simulink model "PositionandSpeedCalculationComponent"  (R2025b)
settings: Solver=FixedStepDiscrete  StartTime=0.0  StopTime=10.0  RelTol=1e-3
settings Model: DataDictionary=TractionEmotorSoftwareArchInterfaceData.sldd  Creator=dakaihu  LastModifiedBy=dakaihu
settings OptimizationCC: ReuseModelBlockBuffer=off
settings RTWCC: GPUComputeCapability=3.5

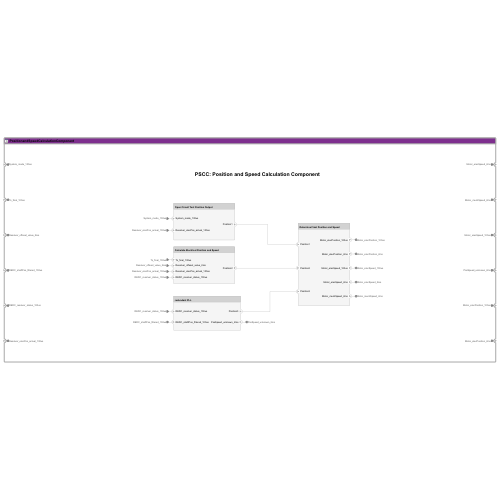
[thumbnail: Simulink's stored preview of the top-level diagram]
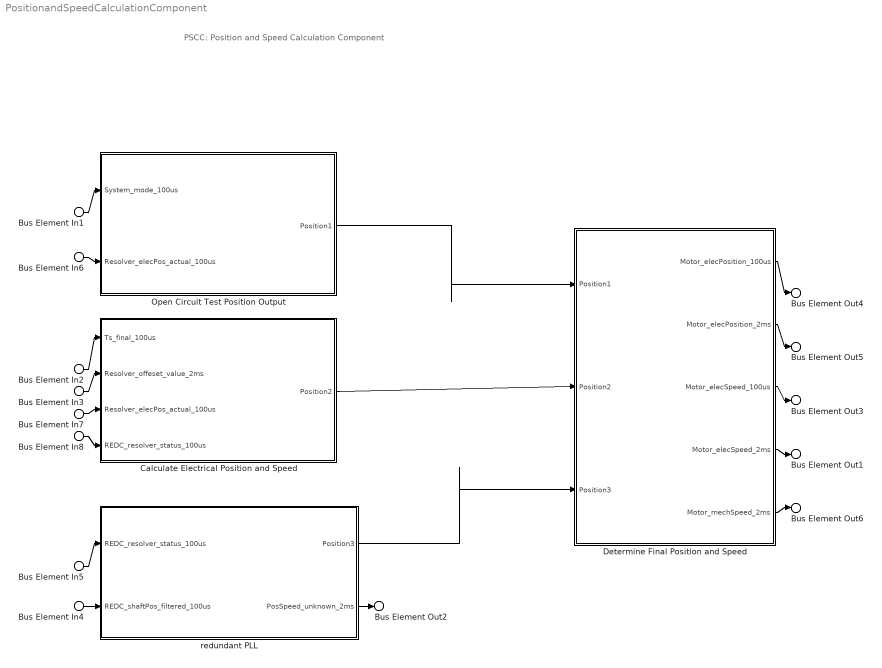
== system PositionandSpeedCalculationComponent ==
  note: PSCC: Position and Speed Calculation Component
  Bus Element In1 : Inport  PortName=System_mode_100us
  Bus Element In2 : Inport  Port=2  PortName=Ts_final_100us
  Bus Element In3 : Inport  Port=3  PortName=Resolver_offeset_value_2ms
  Bus Element In4 : Inport  Port=4  PortName=REDC_shaftPos_filtered_100us
  Bus Element In5 : Inport  Port=5  PortName=REDC_resolver_status_100us
  Bus Element In8 : Inport  Port=5  PortName=REDC_resolver_status_100us
  Bus Element In6 : Inport  Port=6  PortName=Resolver_elecPos_actual_100us
  Bus Element In7 : Inport  Port=6  PortName=Resolver_elecPos_actual_100us
  Calculate Electrical Position and Speed : Subsystem
      settings: PortSchema="{\"entries\":[{\"content\":{\"headerSize\":26,\"margin\":15,\"minimumSpacing\":25,\"sides\":[{\"content\":{\"connectorIds\":[\"In1\",\"In2\",\"In3\",\"In4\"]},\"type\":\"ConnectorPlacement.EquallySpacedRectSide\",\"uuid\":\"b16d0344-473b-4e33-95de-addbcbf18312\"},{\"content\":{\"connectorIds\":[\"Out1\"],\"side\":\"RIGHT\"},\"type\":\"ConnectorPlacement.EquallySpacedRectSide\",\"uuid\":\"7a9166db-696c-4525-87dc-5b08a993a34a\"},{\"content\":{\"connectorIds\":[],\"side\":\"TOP\"},\"type\":\"ConnectorPlacement.EquallySpacedRectSide\",\"uuid\":\"c2a34d16-9517-4bb1-8272-822cdcb4c574\"},{\"content\":{\"connectorIds\":[],\"side\":\"BOTTOM\"},\"type\":\"ConnectorPlacement.EquallySpacedRectSide\",\"uuid\":\"6a225a83-03bd-45b2-94f6-40f1b6cfb673\"}]},\"type\":\"ConnectorPlacement.EquallySpacedConnector\",\"uuid\":\"b21d167c-028b-4471-80b0-68b474506654\"}],\"packageUris\":[\"http://schema.mathworks.com/mf0/Connector/R2020b\"],\"version\":\"1.0\"}"
  Determine Final Position and Speed : Subsystem
      settings: PortSchema="{\"entries\":[{\"content\":{\"headerSize\":26,\"margin\":15,\"minimumSpacing\":25,\"sides\":[{\"content\":{\"connectorIds\":[\"In1\",\"In2\",\"In3\"]},\"type\":\"ConnectorPlacement.EquallySpacedRectSide\",\"uuid\":\"b16d0344-473b-4e33-95de-addbcbf18312\"},{\"content\":{\"connectorIds\":[\"Out1\",\"Out2\",\"Out3\",\"Out4\",\"Out5\"],\"side\":\"RIGHT\"},\"type\":\"ConnectorPlacement.EquallySpacedRectSide\",\"uuid\":\"7a9166db-696c-4525-87dc-5b08a993a34a\"},{\"content\":{\"connectorIds\":[],\"side\":\"TOP\"},\"type\":\"ConnectorPlacement.EquallySpacedRectSide\",\"uuid\":\"c2a34d16-9517-4bb1-8272-822cdcb4c574\"}]},\"type\":\"ConnectorPlacement.EquallySpacedConnector\",\"uuid\":\"b21d167c-028b-4471-80b0-68b474506654\"}],\"packageUris\":[\"http://schema.mathworks.com/mf0/Connector/R2020b\"],\"version\":\"1.0\"}"
  Open Circuit Test Position Output : Subsystem
      settings: PortSchema="{\"entries\":[{\"content\":{\"headerSize\":26,\"margin\":15,\"minimumSpacing\":25,\"sides\":[{\"content\":{\"connectorIds\":[\"In1\",\"In2\"]},\"type\":\"ConnectorPlacement.EquallySpacedRectSide\",\"uuid\":\"b16d0344-473b-4e33-95de-addbcbf18312\"},{\"content\":{\"connectorIds\":[\"Out1\"],\"side\":\"RIGHT\"},\"type\":\"ConnectorPlacement.EquallySpacedRectSide\",\"uuid\":\"7a9166db-696c-4525-87dc-5b08a993a34a\"},{\"content\":{\"connectorIds\":[],\"side\":\"TOP\"},\"type\":\"ConnectorPlacement.EquallySpacedRectSide\",\"uuid\":\"c2a34d16-9517-4bb1-8272-822cdcb4c574\"}]},\"type\":\"ConnectorPlacement.EquallySpacedConnector\",\"uuid\":\"b21d167c-028b-4471-80b0-68b474506654\"}],\"packageUris\":[\"http://schema.mathworks.com/mf0/Connector/R2020b\"],\"version\":\"1.0\"}"
  redundant PLL : Subsystem
      settings: PortSchema="{\"entries\":[{\"content\":{\"headerSize\":26,\"margin\":15,\"minimumSpacing\":25,\"sides\":[{\"content\":{\"connectorIds\":[\"In1\",\"In2\"]},\"type\":\"ConnectorPlacement.EquallySpacedRectSide\",\"uuid\":\"b16d0344-473b-4e33-95de-addbcbf18312\"},{\"content\":{\"connectorIds\":[\"Out1\",\"Out2\"],\"side\":\"RIGHT\"},\"type\":\"ConnectorPlacement.EquallySpacedRectSide\",\"uuid\":\"7a9166db-696c-4525-87dc-5b08a993a34a\"},{\"content\":{\"connectorIds\":[],\"side\":\"TOP\"},\"type\":\"ConnectorPlacement.EquallySpacedRectSide\",\"uuid\":\"c2a34d16-9517-4bb1-8272-822cdcb4c574\"}]},\"type\":\"ConnectorPlacement.EquallySpacedConnector\",\"uuid\":\"b21d167c-028b-4471-80b0-68b474506654\"}],\"packageUris\":[\"http://schema.mathworks.com/mf0/Connector/R2020b\"],\"version\":\"1.0\"}"
  Bus Element Out1 : Outport  PortName=Motor_elecSpeed_2ms
  Bus Element Out6 : Outport  Port=2  PortName=Motor_mechSpeed_2ms
  Bus Element Out3 : Outport  Port=3  PortName=Motor_elecSpeed_100us
  Bus Element Out2 : Outport  Port=4  PortName=PosSpeed_unknown_2ms
  Bus Element Out4 : Outport  Port=5  PortName=Motor_elecPosition_100us
  Bus Element Out5 : Outport  Port=6  PortName=Motor_elecPosition_2ms
  wires:
  Bus Element In1/1 -> Open Circuit Test Position Output/1(System_mode_100us)
  Bus Element In6/1 -> Open Circuit Test Position Output/2(Resolver_elecPos_actual_100us)
  Open Circuit Test Position Output/1(Position1) -> Determine Final Position and Speed/1(Position1)
  Calculate Electrical Position and Speed/1(Position2) -> Determine Final Position and Speed/2(Position2)
  Determine Final Position and Speed/1(Motor_elecPosition_100us) -> Bus Element Out4/1
  Bus Element In5/1 -> redundant PLL/1(REDC_resolver_status_100us)
  Bus Element In2/1 -> Calculate Electrical Position and Speed/1(Ts_final_100us)
  Bus Element In3/1 -> Calculate Electrical Position and Speed/2(Resolver_offeset_value_2ms)
  Bus Element In7/1 -> Calculate Electrical Position and Speed/3(Resolver_elecPos_actual_100us)
  Bus Element In8/1 -> Calculate Electrical Position and Speed/4(REDC_resolver_status_100us)
  Bus Element In4/1 -> redundant PLL/2(REDC_shaftPos_filtered_100us)
  redundant PLL/1(Position3) -> Determine Final Position and Speed/3(Position3)
  Determine Final Position and Speed/3(Motor_elecSpeed_100us) -> Bus Element Out3/1
  Determine Final Position and Speed/2(Motor_elecPosition_2ms) -> Bus Element Out5/1
  Determine Final Position and Speed/4(Motor_elecSpeed_2ms) -> Bus Element Out1/1
  Determine Final Position and Speed/5(Motor_mechSpeed_2ms) -> Bus Element Out6/1
  redundant PLL/2(PosSpeed_unknown_2ms) -> Bus Element Out2/1

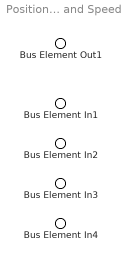
== system PositionandSpeedCalculationComponent/Calculate Electrical Position and Speed ==
  Bus Element In1 : Inport  PortName=Ts_final_100us
  Bus Element In2 : Inport  Port=2  PortName=Resolver_offeset_value_2ms
  Bus Element In3 : Inport  Port=3  PortName=Resolver_elecPos_actual_100us
  Bus Element In4 : Inport  Port=4  PortName=REDC_resolver_status_100us
  Bus Element Out1 : Outport  PortName=Position2

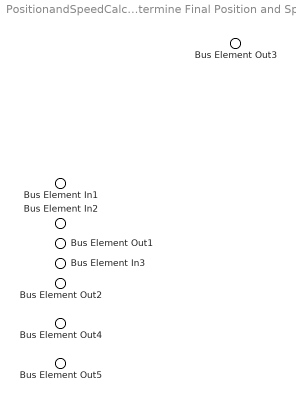
== system PositionandSpeedCalculationComponent/Determine Final Position and Speed ==
  Bus Element In1 : Inport  PortName=Position1
  Bus Element In2 : Inport  Port=2  PortName=Position2
  Bus Element In3 : Inport  Port=3  PortName=Position3
  Bus Element Out1 : Outport  PortName=Motor_elecPosition_100us
  Bus Element Out3 : Outport  Port=2  PortName=Motor_elecPosition_2ms
  Bus Element Out2 : Outport  Port=3  PortName=Motor_elecSpeed_100us
  Bus Element Out4 : Outport  Port=4  PortName=Motor_elecSpeed_2ms
  Bus Element Out5 : Outport  Port=5  PortName=Motor_mechSpeed_2ms

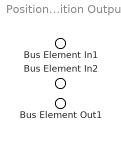
== system PositionandSpeedCalculationComponent/Open Circuit Test Position Output ==
  Bus Element In1 : Inport  PortName=System_mode_100us
  Bus Element In2 : Inport  Port=2  PortName=Resolver_elecPos_actual_100us
  Bus Element Out1 : Outport  PortName=Position1

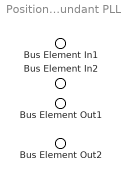
== system PositionandSpeedCalculationComponent/redundant PLL ==
  Bus Element In1 : Inport  PortName=REDC_resolver_status_100us
  Bus Element In2 : Inport  Port=2  PortName=REDC_shaftPos_filtered_100us
  Bus Element Out1 : Outport  PortName=Position3
  Bus Element Out2 : Outport  Port=2  PortName=PosSpeed_unknown_2ms
